simulink model "GFLIB_IntegratorTR_BAM_FLT"  (Simulink 7.3)
settings: Solver=ode45  StartTime=0.0  StopTime=10.0  RelTol=1e-3
undefined symbols (not defined in the file): fltC1
settings Model: Creator=RE004C  LastModifiedBy=RE004C
settings HardwareCC: ProdIntDivRoundTo=Zero  ProdEndianess=BigEndian  ProdHWDeviceType=Freescale->32-bit PowerPC

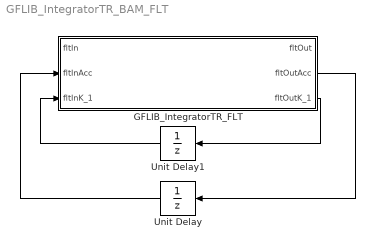
== system GFLIB_IntegratorTR_BAM_FLT ==
  GFLIB_IntegratorTR_FLT : Subsystem  mask(GFLIB_IntegratorTR_FLT){fltC1=fltC1}
      mask help: Bit accurate model of discrete trapezoidal integrator. All parameters as well as input and output are full float range.
      mask init:
      | pos = get_param(gcb, 'Position');width = pos(3) - pos(1); height = pos(4) - pos(2);tX=width/2;tY=height*0.9;
      mask Display:
      | color('black');
      | port_label('input',1,'fltIn');
      | port_label('input',2,'fltInAcc');
      | port_label('input',3,'fltInK_1');
      | port_label('output',1,'fltOut');
      | port_label('output',2,'fltOutAcc');
      | port_label('output',3,'fltOutK_1');
      | color('black');
      | disp('GFLIB_IntegratorTR_FLT');
      | color('blue');
      | text(tX,tY, 'BAM', 'horizontalAlignment', 'center');
  Unit Delay : UnitDelay  SampleTime=-1
  Unit Delay1 : UnitDelay  SampleTime=-1
  wires:
  GFLIB_IntegratorTR_FLT/2(fltOutAcc) -> Unit Delay/1
  Unit Delay/1 -> GFLIB_IntegratorTR_FLT/2(fltInAcc)
  GFLIB_IntegratorTR_FLT/3(fltOutK_1) -> Unit Delay1/1
  Unit Delay1/1 -> GFLIB_IntegratorTR_FLT/3(fltInK_1)

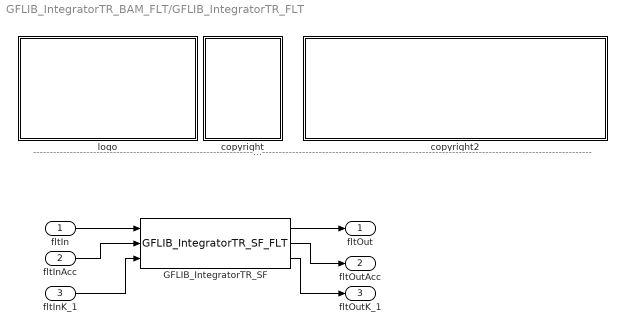
== system GFLIB_IntegratorTR_BAM_FLT/GFLIB_IntegratorTR_FLT ==
  note: ---------------------------------------------------------------------------------------------------------------------------------------------------------------------------------------------------
  fltIn : Inport  OutDataType=fixdt(1, 16)  OutScaling=2^0
  fltInAcc : Inport  Port=2  OutDataType=fixdt(1, 16)  OutScaling=2^0
  fltInK_1 : Inport  Port=3  OutDataType=fixdt(1, 16)  OutScaling=2^0
  GFLIB_IntegratorTR_SF : S-Function  FunctionName=GFLIB_IntegratorTR_SF_FLT  Parameters=fltC1  EnableBusSupport=off
  copyright : Subsystem
      mask Display: text(10,90,'FILE:');text(10,75,'DESRIPTION:')text(10,60,'COPYRIGHT:')text(10,45,'VERSION:')text(10,30,'DATE:')
  copyright2 : Subsystem
      mask Display: text(10,90,'GFLIB_IntegratorTR_BAM_FLT.mdl');text(10,75,'Discrete integrator transformed from linear model using Billinear (trapezoidal) transformation.');text(10,60,'Freescale')text(10,45,'0.1');text(10,30,'16-Jan-2012');
  logo : Subsystem
      mask Display: image(imread('logo.jpg'))
  fltOut : Outport  OutDataType=fixdt(1, 16)  OutScaling=2^0
  fltOutAcc : Outport  Port=2  OutDataType=fixdt(1, 16)  OutScaling=2^0
  fltOutK_1 : Outport  Port=3  OutDataType=fixdt(1, 16)  OutScaling=2^0
  wires:
  fltIn/1 -> GFLIB_IntegratorTR_SF/1
  GFLIB_IntegratorTR_SF/1 -> fltOut/1
  fltInAcc/1 -> GFLIB_IntegratorTR_SF/2
  fltInK_1/1 -> GFLIB_IntegratorTR_SF/3
  GFLIB_IntegratorTR_SF/2 -> fltOutAcc/1
  GFLIB_IntegratorTR_SF/3 -> fltOutK_1/1

== system GFLIB_IntegratorTR_BAM_FLT/GFLIB_IntegratorTR_FLT/copyright ==

== system GFLIB_IntegratorTR_BAM_FLT/GFLIB_IntegratorTR_FLT/copyright2 ==

== system GFLIB_IntegratorTR_BAM_FLT/GFLIB_IntegratorTR_FLT/logo ==
